simulink model "targetingLib"  (R2026b)
settings: Solver=VariableStepAuto
undefined symbols (not defined in the file or in its folder): maxval_sc, minval_sc, modval, samptime, Slope1, Slope2, threshold_add
libraries: hdlsllib x57, simulink x19, simulink_extras x11, dspsigops x2, sl_signal_attributes x2
(part 3 of 3)

== system targetingLib/Energy Detector/Energy Detector/Energy Detector/Signal Detection/Energy Accumulator/ED ACC1/Pow ==
  DataIn : Inport
  Add : Sum
  Complex to Real-Imag : ComplexToRealImag
  Delay{,1..4,7} (6 alike) : Delay  InitialCondition=0  UseCircularBuffer=on
  Delay5 : Delay  DelayLength=1  InitialCondition=0  UseCircularBuffer=on
  Delay6 : Delay  DelayLength=1  InitialCondition=0  UseCircularBuffer=on
  Delay8 : Delay  DelayLength=1  InitialCondition=0  UseCircularBuffer=on
  Mul : Product  Inputs=**
  Mul1 : Product  Inputs=**
  DataOut : Outport
  wires:
  Delay4/1 -> Delay6/1
  Delay8/1 -> DataOut/1
  Delay5/1 -> Add/2
  Delay2/1 -> Mul1/2
  Mul/1 -> Delay4/1
  Delay7/1 -> Delay2/1, Delay3/1
  DataIn/1 -> Complex to Real-Imag/1
  Delay/1 -> Mul/2
  Add/1 -> Delay8/1
  Delay6/1 -> Add/1
  Complex to Real-Imag/2 -> Delay7/1
  Delay1/1 -> Mul/1
  Complex to Real-Imag/1 -> Delay1/1, Delay/1
  Mul1/1 -> Delay5/1
  Delay3/1 -> Mul1/1

== system targetingLib/Energy Detector/Energy Detector/Energy Detector/Signal Detection/Energy Accumulator/ED ACC1/Pow1 ==
  DataIn : Inport
  Add : Sum
  Complex to Real-Imag : ComplexToRealImag
  Delay{,1..4,7} (6 alike) : Delay  InitialCondition=0  UseCircularBuffer=on
  Delay5 : Delay  DelayLength=1  InitialCondition=0  UseCircularBuffer=on
  Delay6 : Delay  DelayLength=1  InitialCondition=0  UseCircularBuffer=on
  Delay8 : Delay  DelayLength=1  InitialCondition=0  UseCircularBuffer=on
  Mul : Product  Inputs=**
  Mul1 : Product  Inputs=**
  DataOut : Outport
  wires:
  Delay4/1 -> Delay6/1
  Delay8/1 -> DataOut/1
  Delay5/1 -> Add/2
  Delay2/1 -> Mul1/2
  Mul/1 -> Delay4/1
  Delay7/1 -> Delay2/1, Delay3/1
  DataIn/1 -> Complex to Real-Imag/1
  Delay/1 -> Mul/2
  Add/1 -> Delay8/1
  Delay6/1 -> Add/1
  Complex to Real-Imag/2 -> Delay7/1
  Delay1/1 -> Mul/1
  Complex to Real-Imag/1 -> Delay1/1, Delay/1
  Mul1/1 -> Delay5/1
  Delay3/1 -> Mul1/1

== system targetingLib/Energy Detector/Energy Detector/Energy Detector/Signal Detection/Energy Accumulator/ED ACC1/WT Accumulator ==
  E : Inport
  R : Inport  Port=2
  DataIn : Inport  Port=3
  InitDataIn : Inport  Port=4
  InitEnb : Inport  Port=5
  AccHigh : Subsystem
  AccLow : Subsystem
  Bit Concat : hdlsllib/Logic and Bit Operations/Bit Concat  numInputs=2
  Bit Slice1 : hdlsllib/Logic and Bit Operations/Bit Slice  lidx=totalBitwidth-1  ridx=lowerBitwidth
  Bit Slice2 : hdlsllib/Logic and Bit Operations/Bit Slice  lidx=lowerBitwidth-1  ridx=0
  Bit Slice4 : hdlsllib/Logic and Bit Operations/Bit Slice  lidx=totalBitwidth-1  ridx=lowerBitwidth
  Bit Slice5 : hdlsllib/Logic and Bit Operations/Bit Slice  lidx=lowerBitwidth-1  ridx=0
  Data Type Propagation : sl_signal_attributes/Data Type Propagation  PropDataType=fixdt(1, 16)  IfRefDouble=double  IfRefSingle=single  IsSigned=IsSigned1  NumBitsBase=NumBits2  NumBitsMult=1  NumBitsAdd=0  NumBitsAllowFinal=-1  PropScaling=2^-10  ValuesUsedBestPrec=[5 -7]  SlopeBase=min([Slope1 Slope2])  SlopeMult=1  SlopeAdd=0  BiasBase=Bias1  BiasMult=1  BiasAdd=0
  Data Type Conversion : DataTypeConversion  ConvertRealWorld=Stored Integer (SI)  SaturateOnIntegerOverflow=off  RndMeth=Floor
  Delay{,1..5} (6 alike) : Delay  DelayLength=1
  DataOut : Outport  VectorParamsAs1DForOutWhenUnconnected=off
  wires:
  R/1 -> AccLow/4(rst), Delay2/1
  E/1 -> AccLow/3(AccEnb), Delay3/1
  Bit Slice1/1 -> Delay1/1
  Delay/1 -> Bit Concat/2
  Data Type Conversion/1 -> DataOut/1, Data Type Propagation/3
  Bit Concat/1 -> Data Type Conversion/1, Data Type Propagation/2
  InitEnb/1 -> AccLow/2(InitEnb), Delay4/1
  Bit Slice4/1 -> Delay5/1
  Delay3/1 -> AccHigh/3(AccEnb)
  Delay2/1 -> AccHigh/4(rst)
  Delay1/1 -> AccHigh/5(DataIn)
  AccLow/1(CarryOut) -> AccHigh/6(Carry)
  AccHigh/1(AccOut) -> Bit Concat/1
  Bit Slice5/1 -> AccLow/1(InitDataL)
  Bit Slice2/1 -> AccLow/5(DataIn)
  Delay4/1 -> AccHigh/2(InitEnb)
  Delay5/1 -> AccHigh/1(InitDataH)
  AccLow/2(AccOut) -> Delay/1
  InitDataIn/1 -> Bit Slice5/1, Bit Slice4/1
  DataIn/1 -> Data Type Propagation/1, Bit Slice1/1, Bit Slice2/1

== system targetingLib/Energy Detector/Energy Detector/Energy Detector/Signal Detection/Energy Accumulator/ED ACC/WT Accumulator/AccHigh ==
  InitDataH : Inport
  InitEnb : Inport  Port=2
  AccEnb : Inport  Port=3
  rst : Inport  Port=4
  DataIn : Inport  Port=5
  Carry : Inport  Port=6
  Sum : Sum  Inputs=+++  OutDataTypeStr=fixdt(0,totalBitwidth-lowerBitwidth,0)  AccumDataTypeStr=fixdt(0,totalBitwidth-lowerBitwidth,0)
  Switch1 : Switch  Criteria=u2 ~= 0  SaturateOnIntegerOverflow=off  InputSameDT=off
  Unit Delay Enabled Resettable Synchronous1 : hdlsllib/Discrete/Unit Delay Enabled Resettable Synchronous  InitialCondition=0.0  SampleTime=-1
  AccOut : Outport
  wires:
  Carry/1 -> Sum/3
  InitEnb/1 -> Switch1/2
  DataIn/1 -> Sum/1
  InitDataH/1 -> Switch1/1
  Unit Delay Enabled Resettable Synchronous1/1 -> Sum/2, AccOut/1
  AccEnb/1 -> Unit Delay Enabled Resettable Synchronous1/2
  rst/1 -> Unit Delay Enabled Resettable Synchronous1/3
  Sum/1 -> Switch1/3
  Switch1/1 -> Unit Delay Enabled Resettable Synchronous1/1

== system targetingLib/Energy Detector/Energy Detector/Energy Detector/Signal Detection/Energy Accumulator/ED ACC/WT Accumulator/AccLow ==
  InitDataL : Inport
  InitEnb : Inport  Port=2
  AccEnb : Inport  Port=3
  rst : Inport  Port=4
  DataIn : Inport  Port=5
  Bit Slice : hdlsllib/Logic and Bit Operations/Bit Slice  lidx=lowerBitwidth  ridx=lowerBitwidth
  Bit Slice3 : hdlsllib/Logic and Bit Operations/Bit Slice  lidx=lowerBitwidth-1  ridx=0
  Sum1 : Sum  Inputs=|++  OutDataTypeStr=fixdt(0,lowerBitwidth+1,0)  AccumDataTypeStr=fixdt(0,lowerBitwidth+1,0)
  Switch : Switch  Criteria=u2 ~= 0  SaturateOnIntegerOverflow=off  InputSameDT=off
  Unit Delay Enabled Resettable Synchronous : hdlsllib/Discrete/Unit Delay Enabled Resettable Synchronous  InitialCondition=0.0  SampleTime=-1
  CarryOut : Outport
  AccOut : Outport  Port=2
  wires:
  Switch/1 -> Unit Delay Enabled Resettable Synchronous/1
  AccEnb/1 -> Unit Delay Enabled Resettable Synchronous/2
  InitEnb/1 -> Switch/2
  Unit Delay Enabled Resettable Synchronous/1 -> Bit Slice/1, Bit Slice3/1
  rst/1 -> Unit Delay Enabled Resettable Synchronous/3
  Sum1/1 -> Switch/3
  InitDataL/1 -> Switch/1
  DataIn/1 -> Sum1/2
  Bit Slice3/1 -> Sum1/1, AccOut/1
  Bit Slice/1 -> CarryOut/1

== system targetingLib/Energy Detector/Energy Detector/Energy Detector/Signal Detection/Energy Accumulator/ED ACC1/WT Accumulator/AccHigh ==
  InitDataH : Inport
  InitEnb : Inport  Port=2
  AccEnb : Inport  Port=3
  rst : Inport  Port=4
  DataIn : Inport  Port=5
  Carry : Inport  Port=6
  Sum : Sum  Inputs=+++  OutDataTypeStr=fixdt(0,totalBitwidth-lowerBitwidth,0)  AccumDataTypeStr=fixdt(0,totalBitwidth-lowerBitwidth,0)
  Switch1 : Switch  Criteria=u2 ~= 0  SaturateOnIntegerOverflow=off  InputSameDT=off
  Unit Delay Enabled Resettable Synchronous1 : hdlsllib/Discrete/Unit Delay Enabled Resettable Synchronous  InitialCondition=0.0  SampleTime=-1
  AccOut : Outport
  wires:
  Carry/1 -> Sum/3
  InitEnb/1 -> Switch1/2
  DataIn/1 -> Sum/1
  InitDataH/1 -> Switch1/1
  Unit Delay Enabled Resettable Synchronous1/1 -> Sum/2, AccOut/1
  AccEnb/1 -> Unit Delay Enabled Resettable Synchronous1/2
  rst/1 -> Unit Delay Enabled Resettable Synchronous1/3
  Sum/1 -> Switch1/3
  Switch1/1 -> Unit Delay Enabled Resettable Synchronous1/1

== system targetingLib/Energy Detector/Energy Detector/Energy Detector/Signal Detection/Energy Accumulator/ED ACC1/WT Accumulator/AccLow ==
  InitDataL : Inport
  InitEnb : Inport  Port=2
  AccEnb : Inport  Port=3
  rst : Inport  Port=4
  DataIn : Inport  Port=5
  Bit Slice : hdlsllib/Logic and Bit Operations/Bit Slice  lidx=lowerBitwidth  ridx=lowerBitwidth
  Bit Slice3 : hdlsllib/Logic and Bit Operations/Bit Slice  lidx=lowerBitwidth-1  ridx=0
  Sum1 : Sum  Inputs=|++  OutDataTypeStr=fixdt(0,lowerBitwidth+1,0)  AccumDataTypeStr=fixdt(0,lowerBitwidth+1,0)
  Switch : Switch  Criteria=u2 ~= 0  SaturateOnIntegerOverflow=off  InputSameDT=off
  Unit Delay Enabled Resettable Synchronous : hdlsllib/Discrete/Unit Delay Enabled Resettable Synchronous  InitialCondition=0.0  SampleTime=-1
  CarryOut : Outport
  AccOut : Outport  Port=2
  wires:
  Switch/1 -> Unit Delay Enabled Resettable Synchronous/1
  AccEnb/1 -> Unit Delay Enabled Resettable Synchronous/2
  InitEnb/1 -> Switch/2
  Unit Delay Enabled Resettable Synchronous/1 -> Bit Slice/1, Bit Slice3/1
  rst/1 -> Unit Delay Enabled Resettable Synchronous/3
  Sum1/1 -> Switch/3
  InitDataL/1 -> Switch/1
  DataIn/1 -> Sum1/2
  Bit Slice3/1 -> Sum1/1, AccOut/1
  Bit Slice/1 -> CarryOut/1

== matlab function targetingLib/Data Packager/MATLAB Function ==
  data: SN_ output; eob_in input; S output; rst input
function [SN_, S] = eob_decrease_state(eob_in, rst)
persistent eob_reg;
persistent eob_state;
if(isempty(eob_reg))
    eob_reg = false;
    eob_state = false;
end

S = eob_state;
SN_ = ~eob_state;

S_next = eob_state || (eob_in && ~eob_reg);

if(rst)
    eob_reg = false;
    eob_state = false;
else
    eob_reg = eob_in;
    eob_state = S_next;
end

== matlab function targetingLib/Prebuffer/Hysteresis Thresholding/Hysteresis Th ==
  data: rst input; th_H input; state_out output; th_L input
function state_out = fcn(rst, th_H, th_L)
%#codegen

HIGH = true;
LOW = false;

persistent state;
if(isempty(state))
    state = LOW;
end

state_out = state;
switch(state)
    case HIGH
        if(th_L)
            state_next = LOW;
        else
            state_next = HIGH;
        end
    case LOW
        if(th_H)
            state_next = HIGH;
        else
            state_next = LOW;
        end
    otherwise
        state_next = LOW;
end

if(rst)
    state = LOW;
else
    state = state_next;
end

== matlab function targetingLib/Data Packager/OutputController ==
  data: data_out output; valid_out output; pop_out output; last output; eob_out output; hasTimeOut output; enb input; count_num output; rst input boolean; data_in input; valid_in input; ready_in input; eob_in input; hasTimeIn input; trigger input; mode input; rec_num input; state_out output; packet_size input uint16; packet_out output
function [data_out, valid_out, pop_out, last, eob_out, hasTimeOut, count_num, state_out, packet_out] = Output_Ctrl(enb, rst, data_in, valid_in, ready_in, eob_in, hasTimeIn, trigger, mode, rec_num, packet_size)
%#codegen
%% @param out
% data_out:    data output
% valid_out:   Valid output data from DUT
% last:        Last signal of each packet
% eob:         end of burst indicator
% count_num:   Current number of samples that send to host
% state_out:   Data packager state
% packet_out:  Current number of samples per packet
%% @param in
% enb:         Data pack enable
% rst:         Reset system to IDLE
% data_in:     Data input
% valid_in:    Valid input
% rec_num:     Number of samples want to transmit to host or DDR in total
% packet_size  Required number of samples per packet

% +---------------+-------------------------------------------+
% | IDLE          | REC            | FINISH                   |
% +---------------+-------------------------------------------+
% | System idle,  | Record a fixed | Current recording        |
% | initial state | number of data | finishes, wait for reset |
% +---------------+-------------------------------------------+
IDLE = ufi(0,3,0);
REC = ufi(1,3,0);
FINISH = ufi(4,3,0);
BURST = false;
CONTINUOUS = true;


persistent state;  % system state register
persistent counter_reg;  % number of recorded samples counter
persistent packet_size_reg;
persistent counter_last_reg;  % number of samples of current recorded packet counter
persistent hasTimeOut_reg;
persistent data_buff eob_buff;
persistent r;
persistent w;
SKID_BUFF_SIZE = 8;  % skid buffer size
BUFF_COUNTER_DEPTH = ceil(log2(SKID_BUFF_SIZE))+1;

if(isempty(state))
    counter_reg = ufi(0,32,0);
    packet_size_reg = ufi(256,16,0);
    counter_last_reg = ufi(0,16,0);
    hasTimeOut_reg = false;
    data_buff = cast(zeros(SKID_BUFF_SIZE,1),'like',data_in);
    eob_buff = cast(zeros(SKID_BUFF_SIZE,1),'like',eob_in);
    state = IDLE;
    r = fi(0,0,BUFF_COUNTER_DEPTH,0,hdlfimath);
    w = fi(0,0,BUFF_COUNTER_DEPTH,0,hdlfimath);
end

state_out = state;
count_num = counter_reg;
packet_out = packet_size_reg;
rs = bitsliceget(r,BUFF_COUNTER_DEPTH-1,1);
ws = bitsliceget(w,BUFF_COUNTER_DEPTH-1,1);
burst_mode = mode == BURST;
continuous_mode = mode == CONTINUOUS;

if(burst_mode)
    valid_in_internal = valid_in;
    rec_finish = counter_reg==rec_num || eob_buff(rs+1);
else
    valid_in_internal = valid_in && ~eob_buff(rs+1);
    rec_finish = eob_buff(rs+1);
end



switch(state)
    case IDLE
        if(valid_in && enb && trigger)
            state_next = REC;
            counter_reg(:) = 1;
            counter_last_reg(:) = 1;
            packet_size_reg(:) = packet_size;
            data_buff(ws+1) = data_in;
            eob_buff(ws+1) = eob_in;
            w(:) = w+1;
            if(hasTimeIn)
                hasTimeOut_reg = true;
            else
                hasTimeOut_reg = false;
            end
        else
            state_next = IDLE;
            w(:) = 0;
            r(:) = 0;
            counter_reg(:) = 0;
            counter_last_reg(:) = 0;
            hasTimeOut_reg = false;
        end
        data_out = data_buff(rs+1);
        valid_out = false;
        last = false;
        eob_out = false;
        hasTimeOut = false;
        pop_out = ready_in;

    case REC
        %% Skid buffer
        if(ready_in && valid_in_internal)
            data_out = data_buff(rs+1);
            r(:) = r + 1;
            data_buff(ws+1) = data_in;
            eob_buff(ws+1) = eob_in;
            w(:) = w+1;
            valid_out_signal = true;
        elseif(~ready_in && valid_in_internal)
            data_out = data_buff(rs+1);
            data_buff(ws+1) = data_in;
            eob_buff(ws+1) = eob_in;
            w(:) = w + 1;
            valid_out_signal = false;
        elseif(ready_in && ~valid_in_internal)
            if(fi(w-r,0,BUFF_COUNTER_DEPTH,0,hdlfimath)~=1)
                data_out = data_buff(rs+1);
                r(:) = r + 1;
                valid_out_signal = true;
            else
                data_out = data_buff(rs+1);
                if(rec_finish)
                    valid_out_signal = true;
                else
                    valid_out_signal = false;
                end
            end
        else
            data_out = data_buff(rs+1);
            valid_out_signal = false;
        end
        %% Data output
        hasTimeOut = hasTimeOut_reg;
        if(rec_finish && valid_out_signal)% finish current record
            valid_out = true;
            last = true;
            eob_out = true;
            state_next = FINISH;
        elseif(valid_out_signal)  % current record not finished
            if(counter_last_reg == packet_size_reg)
                counter_last_reg(:) = 1;
                hasTimeOut_reg = false;
                last = true;
            else
                last = false;
                counter_last_reg(:) = counter_last_reg + 1;
            end
            counter_reg(:) = counter_reg + 1;
            eob_out = false;
            valid_out = true;
            state_next = REC;
        else
            valid_out = false;
            last = false;
            eob_out = false;
            state_next = REC;
        end
        pop_out = ready_in;

    case FINISH
        state_next = FINISH;
        data_out = data_buff(rs+1);
        valid_out = false;
        last = false;
        eob_out = false;
        hasTimeOut = false;
        pop_out = false;
    otherwise
        state_next = IDLE;
        data_out = data_buff(rs+1);
        valid_out = false;
        last = false;
        eob_out = false;
        hasTimeOut = false;
        pop_out = false;
end

if(rst)
    state = IDLE;
    counter_reg(:) = 0;
    counter_last_reg(:) = 0;
    data_buff(:) = 0;
    eob_buff(:) = 0;
    w(:) = 0;
    r(:) = 0;
    hasTimeOut_reg = false;
else
    state = state_next;
end

%%sub functions

== matlab function targetingLib/Energy Detector/Energy Detector/Energy Detector/Signal Detection/Dual Delayer/Variable Delayer0/delay_line_ctrl ==
  settings: fimath=fimath('OverflowAction', 'Wrap', 'RoundingMethod','Nearest');
  data: addr_out output; init0_c output; valid_out output; delay_length input; de0 input; valid_in input; rst input; depth parameter; n_init_assert output; acc_init output
function [addr_out, init0_c, valid_out, n_init_assert, acc_init]  = delay_line_controller(delay_length, de0, valid_in, rst, depth)
%#codegen
persistent state;
persistent counter_reg;
IDLE = ufi(0,2,0);
INIT = ufi(1,2,0);
DELAY = ufi(2,2,0);

if(isempty(counter_reg))
    counter_reg = ufi(1,depth,0);
end
if(isempty(state))
    state = IDLE;
end

addr_out = counter_reg;
valid_out = valid_in;
switch(state)
    case IDLE
        if(valid_in && ~rst)
            if(de0)
                n_init_assert = true;
                init0_c = false;
                state_next = DELAY;
            else
                n_init_assert = false;
                init0_c = true;
                state_next = INIT;
                counter_reg(:) = 1;
            end
            acc_init = true;
        else
            init0_c = false;
            acc_init = false;
            state_next = IDLE;
            n_init_assert = false;
        end

    case INIT
        if(valid_in)
            if(counter_reg == delay_length)
                init0_c = false;
                n_init_assert = true;
                state_next = DELAY;
            else
                counter_reg(:) = counter_reg + 1;
                init0_c = true;
                n_init_assert = false;
                state_next = INIT;
            end
        else
            init0_c = true;
            n_init_assert = false;
            state_next = INIT;
        end
        acc_init = false;

    case DELAY
        n_init_assert = true;
        init0_c = false;
        state_next = DELAY;
        acc_init = false;

    otherwise
        n_init_assert = false;
        init0_c = true;
        acc_init = false;
        state_next = INIT;
end
if(rst)
    state = IDLE;
    counter_reg(:) = 0;
else
    state = state_next;
end

== matlab function targetingLib/Energy Detector/Energy Detector/Energy Detector/Signal Detection/Dual Delayer/Variable Delayer1/delay_line_ctrl ==
  settings: fimath=fimath('OverflowAction', 'Wrap', 'RoundingMethod','Nearest');
  data: addr_out output; init0_c output; valid_out output; delay_length input; de0 input; valid_in input; rst input; depth parameter; n_init_assert output; acc_init output
function [addr_out, init0_c, valid_out, n_init_assert, acc_init]  = delay_line_controller(delay_length, de0, valid_in, rst, depth)
%#codegen
persistent state;
persistent counter_reg;
IDLE = ufi(0,2,0);
INIT = ufi(1,2,0);
DELAY = ufi(2,2,0);

if(isempty(counter_reg))
    counter_reg = ufi(1,depth,0);
end
if(isempty(state))
    state = IDLE;
end

addr_out = counter_reg;
valid_out = valid_in;
switch(state)
    case IDLE
        if(valid_in && ~rst)
            if(de0)
                n_init_assert = true;
                init0_c = false;
                state_next = DELAY;
            else
                n_init_assert = false;
                init0_c = true;
                state_next = INIT;
                counter_reg(:) = 1;
            end
            acc_init = true;
        else
            init0_c = false;
            acc_init = false;
            state_next = IDLE;
            n_init_assert = false;
        end

    case INIT
        if(valid_in)
            if(counter_reg == delay_length)
                init0_c = false;
                n_init_assert = true;
                state_next = DELAY;
            else
                counter_reg(:) = counter_reg + 1;
                init0_c = true;
                n_init_assert = false;
                state_next = INIT;
            end
        else
            init0_c = true;
            n_init_assert = false;
            state_next = INIT;
        end
        acc_init = false;

    case DELAY
        n_init_assert = true;
        init0_c = false;
        state_next = DELAY;
        acc_init = false;

    otherwise
        n_init_assert = false;
        init0_c = true;
        acc_init = false;
        state_next = INIT;
end
if(rst)
    state = IDLE;
    counter_reg(:) = 0;
else
    state = state_next;
end
